simulink model "simulation_impulse"  (R2023b)
settings: Solver=VariableStepAuto  StartTime=0.0  StopTime=10.0  RelTol=1e-3
InitFcn:
  | param = plant_param();
  | sysc = plant_sysc(param,option);
values from neighbouring files (symbols this model uses):
  option = struct("qe",0)    [plot_bode.m]
undefined symbols (not defined in the file or in its folder): x0
settings Model: Creator=block  LastModifiedBy=block

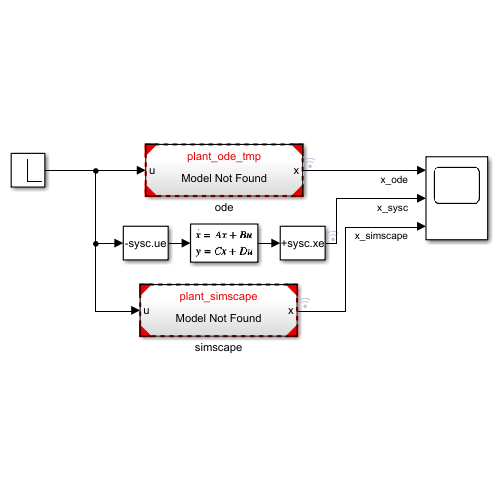
[thumbnail: Simulink's stored preview of the top-level diagram]
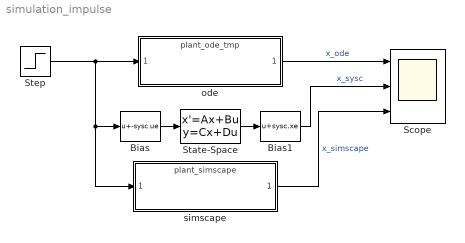
== system simulation_impulse ==
  Bias : Bias  Bias=-sysc.ue  SaturateOnIntegerOverflow=off
  Bias1 : Bias  Bias=sysc.xe  SaturateOnIntegerOverflow=off
  Scope : Scope  NumInputPorts=3
  State-Space : StateSpace  A=sysc.A  B=sysc.B  C=sysc.C  D=sysc.D  InitialCondition=x0-sysc.xe
  Step : Step  Time=0.01  Before=100  After=0  SampleTime=0
  ode : ModelReference  ModelNameDialog=plant_ode_tmp  SimulationMode=Normal  ModelReferenceVersion=1.40
  simscape : ModelReference  ModelNameDialog=plant_simscape  SimulationMode=Normal  ModelReferenceVersion=1.40
  wires:
  Bias1/1 -> Scope/2  "x_sysc"
  ode/1 -> Scope/1  "x_ode"
  Step/1 -> simscape/1, Bias/1, ode/1
  simscape/1 -> Scope/3  "x_simscape"
  Bias/1 -> State-Space/1
  State-Space/1 -> Bias1/1
